simulink model "Compressor_Simulation"  (R2019b)
settings: Solver=FixedStepDiscrete  StartTime=0.0  StopTime=inf  RelTol=1e-3
libraries: dspsrcs4 x3, audiodynamicrange x1
settings Model: Creator=Josh  LastModifiedBy=Josh
settings SolverCC: AutoInsertRateTranBlk=on
settings DataIOCC: LimitDataPoints=on  SaveOutput=off  SignalLogging=off  SaveTime=off
settings OptimizationCC: LifeSpan=inf  SimCompilerOptimization=on
settings DebuggingCC: AlgebraicLoopMsg=error  SingleTaskRateTransMsg=error  AllowSymbolicDim=off  SFUnexpectedBacktrackingDiag=warning  SFNoUnconditionalDefaultTransitionDiag=warning  SFExecutionAtInitializationDiag=none  ArithmeticOperatorsInVariantConditions=warning
settings SFSimCC: SimUseLocalCustomCode=off  CustomCodeUndefinedFunction=UseInterfaceOnly
settings RTWCC: RTWUseLocalCustomCode=off
settings CodeAppCC: StateflowObjectComments=on
settings GRTTargetCC: TargetLangStandard=C89/C90 (ANSI)  GeneratePreprocessorConditionals=Disable all
settings ConfigComp: CovMetricSettings=dw  CovHtmlReporting=on  CovSaveCumulativeToWorkspaceVar=on  CovSaveSingleToWorkspaceVar=on  CovExternalEMLEnable=off  CovSFcnEnable=off

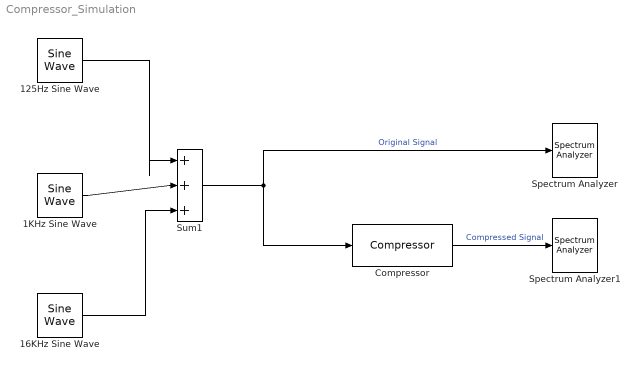
== system Compressor_Simulation ==
  125Hz Sine Wave : dspsrcs4/Sine Wave  Amplitude=1  Frequency=125  Phase=0  SampleMode=Discrete  OutComplex=Real  CompMethod=Trigonometric fcn  TableSize=Speed  SampleTime=1/44100  SamplesPerFrame=256  ResetState=Restart at time zero  OutputFrames=off  dataType=double  wordLen=16  udDataType=sfix(16)  fracBitsMode=Best precision  numFracBits=15  OutDataTypeStr=double  LastOutDataTypeStr=double
  16KHz Sine Wave : dspsrcs4/Sine Wave  Amplitude=5  Frequency=16000  Phase=0  SampleMode=Discrete  OutComplex=Real  CompMethod=Trigonometric fcn  TableSize=Speed  SampleTime=1/44100  SamplesPerFrame=256  ResetState=Restart at time zero  OutputFrames=off  dataType=double  wordLen=16  udDataType=sfix(16)  fracBitsMode=Best precision  numFracBits=15  OutDataTypeStr=double  LastOutDataTypeStr=double
  1KHz Sine Wave : dspsrcs4/Sine Wave  Amplitude=15  Frequency=1000  Phase=0  SampleMode=Discrete  OutComplex=Real  CompMethod=Trigonometric fcn  TableSize=Speed  SampleTime=1/44100  SamplesPerFrame=256  ResetState=Restart at time zero  OutputFrames=off  dataType=double  wordLen=16  udDataType=sfix(16)  fracBitsMode=Best precision  numFracBits=15  OutDataTypeStr=double  LastOutDataTypeStr=double
  Compressor : audiodynamicrange/Compressor  ThresholdPort=off  Threshold=-50.0  RatioPort=off  Ratio=5.0  KneeWidthPort=off  KneeWidth=0.0  AttackTimePort=off  AttackTime=0.05  ReleaseTimePort=off  ReleaseTime=0.2  MakeUpGainMode=Property  MakeUpGain=24.0  InheritSampleRate=on  SampleRate=44100  outputGain=off  SimulateUsing=Code generation
      settings: SourceProductName=Audio Toolbox  SourceProductBaseCode=AU
  Spectrum Analyzer : SpectrumAnalyzer
  Spectrum Analyzer1 : SpectrumAnalyzer
  Sum1 : Sum  Inputs=|+++
  wires:
  125Hz Sine Wave/1 -> Sum1/1
  1KHz Sine Wave/1 -> Sum1/2
  Sum1/1 -> Compressor/1, Spectrum Analyzer/1  "Original Signal"
  16KHz Sine Wave/1 -> Sum1/3
  Compressor/1 -> Spectrum Analyzer1/1  "Compressed Signal"
